simulink subsystem "aerodynamics"  (R2024b)
settings: Solver=VariableStepAuto  StartTime=0.0  StopTime=10.0  RelTol=1e-3
undefined symbols (not defined in the file): aero1d__ca0__mach, aero1d__ca0b__mach, aero1d__cad__mach, aero1d__cllp__mach, aero1d__clmq__mach, aero1d__clnr__mach, aero3d__caa__mach__alpha__beta, aero3d__cll0__mach__alpha__beta, aero3d__clldp__mach__alpha__beta, aero3d__clm0__mach__alpha__beta, aero3d__clmdq__mach__alpha__beta, aero3d__cln0__mach__alpha__beta, aero3d__clndr__mach__alpha__beta, aero3d__cn0__mach__alpha__beta, aero3d__cndq__mach__alpha__beta, aero3d__cy0__mach__alpha__beta, aero3d__cydr__mach__alpha__beta, alpha_grid, beta_grid, mach_grid, refa, refl, xcg_ref
settings Model: Creator=yagiz  LastModifiedBy=yagiz

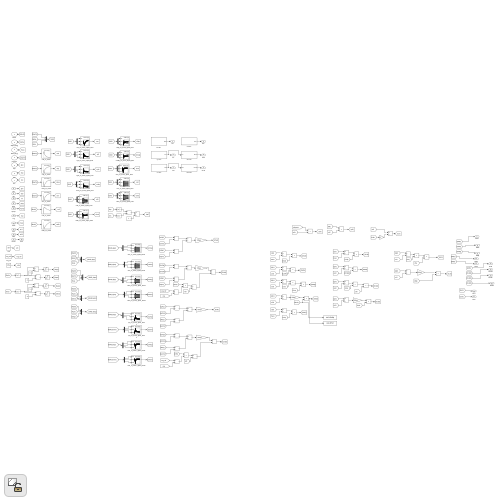
[thumbnail: Simulink's stored preview of the top-level diagram]
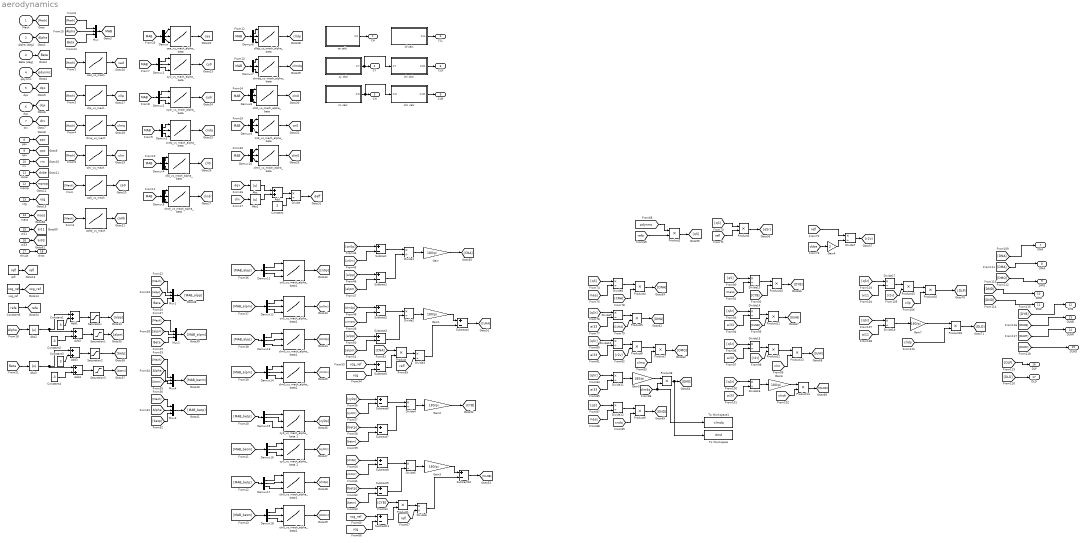
== system aerodynamics ==
  Mach : Inport
  Alpha [deg] : Inport  Port=2
  Beta [deg] : Inport  Port=3
  pdynmc : Inport  Port=4
  dpx : Inport  Port=5
  dqx : Inport  Port=6
  drx : Inport  Port=7
  ppx : Inport  Port=8
  qqx : Inport  Port=9
  rrx : Inport  Port=10
  dvbe : Inport  Port=11
  mprop : Inport  Port=12
  xcg : Inport  Port=13
  mass : Inport  Port=14
  ai11 : Inport  Port=15
  ai33 : Inport  Port=16
  thrust : Inport  Port=17
  Abs{,1..3} (4 alike) : Abs  SaturateOnIntegerOverflow=off
  Add{,1..4} (5 alike) : Sum
  Constant : Constant  Value=2
  Constant1 : Constant  Value=3
  Constant2 : Constant  Value=-3
  Constant3 : Constant  Value=3
  Constant4 : Constant  Value=-3
  Constant6 : Constant  Value=refa
  Demux{,1..18} (19 alike) : Demux  Outputs=3
  Divide{,1..18} (19 alike) : Product  Inputs=*/
  Gain{,1..3,5..7} (7 alike) : Gain  Gain=180/pi
  Gain4 : Gain  Gain=2
  Mux{,1..4} (5 alike) : Mux  Inputs=3
  Product{,1..16,18} (18 alike) : Product
  Saturation : Saturate  UpperLimit=inf  LowerLimit=3
  Saturation1 : Saturate  UpperLimit=inf  LowerLimit=0
  Saturation2 : Saturate  UpperLimit=inf  LowerLimit=3
  Saturation3 : Saturate  UpperLimit=inf  LowerLimit=0
  Subtract{,1..11} (12 alike) : Sum  Inputs=+-
  To Workspace : ToWorkspace  VariableName=dmd  SaveFormat=Timeseries  SampleTime=-1
  To Workspace1 : ToWorkspace  VariableName=clmdq  SaveFormat=Timeseries  SampleTime=-1
  ca calc : Subsystem
  ca0_vs_mach : Lookup_n-D  NumberOfTableDimensions=1  BreakpointsForDimension1=mach_grid  Table=aero1d__ca0__mach  InternalRulePriority=Speed  RndMeth=Simplest
  ca0b_vs_mach : Lookup_n-D  NumberOfTableDimensions=1  BreakpointsForDimension1=mach_grid  Table=aero1d__ca0b__mach  InternalRulePriority=Speed  RndMeth=Simplest
  caa_vs_mach_alpha_beta : Lookup_n-D  NumberOfTableDimensions=3  BreakpointsForDimension1=mach_grid  BreakpointsForDimension2=alpha_grid  BreakpointsForDimension3=beta_grid  Table=aero3d__caa__mach__alpha__beta  InternalRulePriority=Speed  RndMeth=Simplest
      settings: InputPortMap=u0,u1,u2
  cad_vs_mach : Lookup_n-D  NumberOfTableDimensions=1  BreakpointsForDimension1=mach_grid  Table=aero1d__cad__mach  InternalRulePriority=Speed  RndMeth=Simplest
  cll calc : Subsystem
  cll0_vs_mach_alpha_beta : Lookup_n-D  NumberOfTableDimensions=3  BreakpointsForDimension1=mach_grid  BreakpointsForDimension2=alpha_grid  BreakpointsForDimension3=beta_grid  Table=aero3d__cll0__mach__alpha__beta  InternalRulePriority=Speed  RndMeth=Simplest
      settings: InputPortMap=u0,u1,u2
  clldp_vs_mach_alpha_beta : Lookup_n-D  NumberOfTableDimensions=3  BreakpointsForDimension1=mach_grid  BreakpointsForDimension2=alpha_grid  BreakpointsForDimension3=beta_grid  Table=aero3d__clldp__mach__alpha__beta  InternalRulePriority=Speed  RndMeth=Simplest
      settings: InputPortMap=u0,u1,u2
  cllp_vs_mach : Lookup_n-D  NumberOfTableDimensions=1  BreakpointsForDimension1=mach_grid  Table=aero1d__cllp__mach  InternalRulePriority=Speed  RndMeth=Simplest
  clm calc : Subsystem
  clm0_vs_mach_alpha_beta : Lookup_n-D  NumberOfTableDimensions=3  BreakpointsForDimension1=mach_grid  BreakpointsForDimension2=alpha_grid  BreakpointsForDimension3=beta_grid  Table=aero3d__clm0__mach__alpha__beta  InternalRulePriority=Speed  RndMeth=Simplest
      settings: InputPortMap=u0,u1,u2
  clm0_vs_mach_alpha_beta1 : Lookup_n-D  NumberOfTableDimensions=3  BreakpointsForDimension1=mach_grid  BreakpointsForDimension2=alpha_grid  BreakpointsForDimension3=beta_grid  Table=aero3d__clm0__mach__alpha__beta  InternalRulePriority=Speed  RndMeth=Simplest
      settings: InputPortMap=u0,u1,u2
  clm0_vs_mach_alpha_beta2 : Lookup_n-D  NumberOfTableDimensions=3  BreakpointsForDimension1=mach_grid  BreakpointsForDimension2=alpha_grid  BreakpointsForDimension3=beta_grid  Table=aero3d__clm0__mach__alpha__beta  InternalRulePriority=Speed  RndMeth=Simplest
      settings: InputPortMap=u0,u1,u2
  clmdq_vs_mach_alpha_beta : Lookup_n-D  NumberOfTableDimensions=3  BreakpointsForDimension1=mach_grid  BreakpointsForDimension2=alpha_grid  BreakpointsForDimension3=beta_grid  Table=aero3d__clmdq__mach__alpha__beta  InternalRulePriority=Speed  RndMeth=Simplest
      settings: InputPortMap=u0,u1,u2
  clmq_vs_mach : Lookup_n-D  NumberOfTableDimensions=1  BreakpointsForDimension1=mach_grid  Table=aero1d__clmq__mach  InternalRulePriority=Speed  RndMeth=Simplest
  cln calc : Subsystem
  cln0_vs_mach_alpha_beta : Lookup_n-D  NumberOfTableDimensions=3  BreakpointsForDimension1=mach_grid  BreakpointsForDimension2=alpha_grid  BreakpointsForDimension3=beta_grid  Table=aero3d__cln0__mach__alpha__beta  InternalRulePriority=Speed  RndMeth=Simplest
      settings: InputPortMap=u0,u1,u2
  cln0_vs_mach_alpha_beta1 : Lookup_n-D  NumberOfTableDimensions=3  BreakpointsForDimension1=mach_grid  BreakpointsForDimension2=alpha_grid  BreakpointsForDimension3=beta_grid  Table=aero3d__cln0__mach__alpha__beta  InternalRulePriority=Speed  RndMeth=Simplest
      settings: InputPortMap=u0,u1,u2
  cln0_vs_mach_alpha_beta2 : Lookup_n-D  NumberOfTableDimensions=3  BreakpointsForDimension1=mach_grid  BreakpointsForDimension2=alpha_grid  BreakpointsForDimension3=beta_grid  Table=aero3d__cln0__mach__alpha__beta  InternalRulePriority=Speed  RndMeth=Simplest
      settings: InputPortMap=u0,u1,u2
  "clndr_vs_mach_alpha_beta " : Lookup_n-D  NumberOfTableDimensions=3  BreakpointsForDimension1=mach_grid  BreakpointsForDimension2=alpha_grid  BreakpointsForDimension3=beta_grid  Table=aero3d__clndr__mach__alpha__beta  InternalRulePriority=Speed  RndMeth=Simplest
      settings: InputPortMap=u0,u1,u2
  clnr_vs_mach : Lookup_n-D  NumberOfTableDimensions=1  BreakpointsForDimension1=mach_grid  Table=aero1d__clnr__mach  InternalRulePriority=Speed  RndMeth=Simplest
  cn calc : Subsystem
  cn0_vs_mach_alpha_beta : Lookup_n-D  NumberOfTableDimensions=3  BreakpointsForDimension1=mach_grid  BreakpointsForDimension2=alpha_grid  BreakpointsForDimension3=beta_grid  Table=aero3d__cn0__mach__alpha__beta  InternalRulePriority=Speed  RndMeth=Simplest
      settings: InputPortMap=u0,u1,u2
  cn0_vs_mach_alpha_beta1 : Lookup_n-D  NumberOfTableDimensions=3  BreakpointsForDimension1=mach_grid  BreakpointsForDimension2=alpha_grid  BreakpointsForDimension3=beta_grid  Table=aero3d__cn0__mach__alpha__beta  InternalRulePriority=Speed  RndMeth=Simplest
      settings: InputPortMap=u0,u1,u2
  cn0_vs_mach_alpha_beta2 : Lookup_n-D  NumberOfTableDimensions=3  BreakpointsForDimension1=mach_grid  BreakpointsForDimension2=alpha_grid  BreakpointsForDimension3=beta_grid  Table=aero3d__cn0__mach__alpha__beta  InternalRulePriority=Speed  RndMeth=Simplest
      settings: InputPortMap=u0,u1,u2
  cndq_vs_mach_alpha_beta : Lookup_n-D  NumberOfTableDimensions=3  BreakpointsForDimension1=mach_grid  BreakpointsForDimension2=alpha_grid  BreakpointsForDimension3=beta_grid  Table=aero3d__cndq__mach__alpha__beta  InternalRulePriority=Speed  RndMeth=Simplest
      settings: InputPortMap=u0,u1,u2
  cy calc : Subsystem
  "cy0_vs_mach_alpha_beta " : Lookup_n-D  NumberOfTableDimensions=3  BreakpointsForDimension1=mach_grid  BreakpointsForDimension2=alpha_grid  BreakpointsForDimension3=beta_grid  Table=aero3d__cy0__mach__alpha__beta  InternalRulePriority=Speed  RndMeth=Simplest
      settings: InputPortMap=u0,u1,u2
  cy0_vs_mach_alpha_beta 1 : Lookup_n-D  NumberOfTableDimensions=3  BreakpointsForDimension1=mach_grid  BreakpointsForDimension2=alpha_grid  BreakpointsForDimension3=beta_grid  Table=aero3d__cy0__mach__alpha__beta  InternalRulePriority=Speed  RndMeth=Simplest
      settings: InputPortMap=u0,u1,u2
  cy0_vs_mach_alpha_beta 2 : Lookup_n-D  NumberOfTableDimensions=3  BreakpointsForDimension1=mach_grid  BreakpointsForDimension2=alpha_grid  BreakpointsForDimension3=beta_grid  Table=aero3d__cy0__mach__alpha__beta  InternalRulePriority=Speed  RndMeth=Simplest
      settings: InputPortMap=u0,u1,u2
  cydr_vs_mach_alpha_beta : Lookup_n-D  NumberOfTableDimensions=3  BreakpointsForDimension1=mach_grid  BreakpointsForDimension2=alpha_grid  BreakpointsForDimension3=beta_grid  Table=aero3d__cydr__mach__alpha__beta  InternalRulePriority=Speed  RndMeth=Simplest
      settings: InputPortMap=u0,u1,u2
  refl : Constant  Value=refl
  xcg_ref : Constant  Value=xcg_ref
  CA : Outport
  CY : Outport  Port=2
  CN : Outport  Port=3
  CLL : Outport  Port=4
  CLM : Outport  Port=5
  CLN : Outport  Port=6
  DNA : Outport  Port=7
  DMA : Outport  Port=8
  DMQ : Outport  Port=9
  DMD : Outport  Port=10
  DND : Outport  Port=11
  DYB : Outport  Port=12
  DLNB : Outport  Port=13
  DLNR : Outport  Port=14
  DLND : Outport  Port=15
  DLP : Outport  Port=16
  DLD : Outport  Port=17
  thrst : Outport  Port=18
  tag scope: Alpha=global, Beta=global, MAB=global, ai11=global, ai33=global, ca0=global, ca0b=global, caa=global, cad=global, cll0=global, clldp=global, cllp=global, clm0=global, clmdq=global, clmq=global, cln0=global, clndr=global, clnr=global, cn0=global, cndq=global, cy0=global, cydr=global, deff=global, dpx=global, dqx=global, drx=global, dvbe=global, mass=global, mprop=global, pdynmc=global, ppx=global, qqx=global, refa=global, refl=global, rrx=global, xcg=global, xcg_ref=global
  wires:
  Mach/1 -> [Mach]
  Alpha [deg]/1 -> [Alpha]
  Beta [deg]/1 -> [Beta]
  [Mach] -> ca0_vs_mach/1
  [Mach] -> ca0b_vs_mach/1
  [Mach] -> cad_vs_mach/1
  [Mach] -> cllp_vs_mach/1
  [Mach] -> clmq_vs_mach/1
  [Mach] -> clnr_vs_mach/1
  [Alpha] -> Mux/2
  [Mach] -> Mux/1
  [Beta] -> Mux/3
  Mux/1 -> [MAB]
  [MAB] -> Demux/1
  Demux/1 -> caa_vs_mach_alpha_beta/1
  Demux/2 -> caa_vs_mach_alpha_beta/2
  Demux/3 -> caa_vs_mach_alpha_beta/3
  [MAB] -> Demux1/1
  Demux1/2 -> "cy0_vs_mach_alpha_beta "/2
  Demux1/1 -> "cy0_vs_mach_alpha_beta "/1
  Demux1/3 -> "cy0_vs_mach_alpha_beta "/3
  [MAB] -> Demux2/1
  Demux2/2 -> cydr_vs_mach_alpha_beta/2
  Demux2/1 -> cydr_vs_mach_alpha_beta/1
  Demux2/3 -> cydr_vs_mach_alpha_beta/3
  [MAB] -> Demux3/1
  Demux3/2 -> cndq_vs_mach_alpha_beta/2
  Demux3/1 -> cndq_vs_mach_alpha_beta/1
  Demux3/3 -> cndq_vs_mach_alpha_beta/3
  [MAB] -> Demux4/1
  Demux4/2 -> cll0_vs_mach_alpha_beta/2
  Demux4/1 -> cll0_vs_mach_alpha_beta/1
  Demux4/3 -> cll0_vs_mach_alpha_beta/3
  [MAB] -> Demux5/1
  Demux5/2 -> "clndr_vs_mach_alpha_beta "/2
  Demux5/1 -> "clndr_vs_mach_alpha_beta "/1
  Demux5/3 -> "clndr_vs_mach_alpha_beta "/3
  [MAB] -> Demux6/1
  Demux6/2 -> clldp_vs_mach_alpha_beta/2
  Demux6/1 -> clldp_vs_mach_alpha_beta/1
  Demux6/3 -> clldp_vs_mach_alpha_beta/3
  [MAB] -> Demux7/1
  Demux7/2 -> clmdq_vs_mach_alpha_beta/2
  Demux7/1 -> clmdq_vs_mach_alpha_beta/1
  Demux7/3 -> clmdq_vs_mach_alpha_beta/3
  [MAB] -> Demux8/1
  Demux8/2 -> cln0_vs_mach_alpha_beta/2
  Demux8/1 -> cln0_vs_mach_alpha_beta/1
  Demux8/3 -> cln0_vs_mach_alpha_beta/3
  pdynmc/1 -> [pdynmc]
  dpx/1 -> [dpx]
  dqx/1 -> [dqx]
  drx/1 -> [drx]
  qqx/1 -> [qqx]
  ppx/1 -> [ppx]
  rrx/1 -> [rrx]
  dvbe/1 -> [dvbe]
  mprop/1 -> [mprop]
  refl/1 -> [refl]
  xcg_ref/1 -> [xcg_ref]
  xcg/1 -> [xcg]
  cad_vs_mach/1 -> [cad]
  cllp_vs_mach/1 -> [cllp]
  clmq_vs_mach/1 -> [clmq]
  clnr_vs_mach/1 -> [clnr]
  ca0_vs_mach/1 -> [ca0]
  ca0b_vs_mach/1 -> [ca0b]
  caa_vs_mach_alpha_beta/1 -> [caa]
  "cy0_vs_mach_alpha_beta "/1 -> [cy0]
  cydr_vs_mach_alpha_beta/1 -> [cydr]
  cndq_vs_mach_alpha_beta/1 -> [cndq]
  cll0_vs_mach_alpha_beta/1 -> [cll0]
  "clndr_vs_mach_alpha_beta "/1 -> [clndr]
  clldp_vs_mach_alpha_beta/1 -> [clldp]
  clmdq_vs_mach_alpha_beta/1 -> [clmdq]
  cln0_vs_mach_alpha_beta/1 -> [cln0]
  [dqx] -> Abs/1
  Abs/1 -> Add/1
  Abs1/1 -> Add/2
  [drx] -> Abs1/1
  Add/1 -> Divide/1
  Constant/1 -> Divide/2
  Divide/1 -> [deff]
  [MAB] -> Demux9/1
  Demux9/2 -> cn0_vs_mach_alpha_beta/2
  cn0_vs_mach_alpha_beta/1 -> [cn0]
  Demux9/1 -> cn0_vs_mach_alpha_beta/1
  Demux9/3 -> cn0_vs_mach_alpha_beta/3
  Demux10/2 -> clm0_vs_mach_alpha_beta/2
  clm0_vs_mach_alpha_beta/1 -> [clm0]
  Demux10/3 -> clm0_vs_mach_alpha_beta/3
  Demux10/1 -> clm0_vs_mach_alpha_beta/1
  [MAB] -> Demux10/1
  ca calc/1(CA) -> CA/1
  cy calc/1(CY) -> cln calc/1(CY), CY/1
  cn calc/1(CN) -> clm calc/1(CN), CN/1
  cll calc/1(CLL) -> CLL/1
  clm calc/1(CLM) -> CLM/1
  cln calc/1(CLN) -> CLN/1
  [Alpha] -> Abs2/1
  Abs2/1 -> Add2/1, Add1/1
  Constant1/1 -> Add1/2
  Add1/1 -> Saturation/1
  Saturation/1 -> [alpp]
  Add2/1 -> Saturation1/1
  Saturation1/1 -> [alpm]
  Constant2/1 -> Add2/2
  [Beta] -> Abs3/1
  Saturation2/1 -> [betp]
  Add3/1 -> Saturation2/1
  Abs3/1 -> Add4/1, Add3/1
  Saturation3/1 -> [betm]
  Add4/1 -> Saturation3/1
  Constant4/1 -> Add4/2
  Constant3/1 -> Add3/2
  [Mach] -> Mux1/1
  [alpp] -> Mux1/2
  [Beta] -> Mux1/3
  [Beta] -> Mux2/3
  [Mach] -> Mux2/1
  [alpm] -> Mux2/2
  [betp] -> Mux3/3
  [Mach] -> Mux3/1
  [Alpha] -> Mux3/2
  [Mach] -> Mux4/1
  [Alpha] -> Mux4/2
  [betm] -> Mux4/3
  Mux1/1 -> [MAB_alpp]
  Mux2/1 -> [MAB_alpm]
  Mux4/1 -> [MAB_betm]
  Mux3/1 -> [MAB_betp]
  [MAB_alpp] -> Demux11/1
  Demux11/1 -> cn0_vs_mach_alpha_beta1/1
  Demux11/2 -> cn0_vs_mach_alpha_beta1/2
  Demux11/3 -> cn0_vs_mach_alpha_beta1/3
  Demux12/1 -> cn0_vs_mach_alpha_beta2/1
  Demux12/2 -> cn0_vs_mach_alpha_beta2/2
  [MAB_alpm] -> Demux12/1
  Demux12/3 -> cn0_vs_mach_alpha_beta2/3
  Demux14/1 -> clm0_vs_mach_alpha_beta2/1
  Demux13/1 -> clm0_vs_mach_alpha_beta1/1
  Demux13/2 -> clm0_vs_mach_alpha_beta1/2
  Demux14/3 -> clm0_vs_mach_alpha_beta2/3
  [MAB_alpm] -> Demux14/1
  Demux14/2 -> clm0_vs_mach_alpha_beta2/2
  [MAB_alpp] -> Demux13/1
  Demux13/3 -> clm0_vs_mach_alpha_beta1/3
  cn0_vs_mach_alpha_beta1/1 -> [cn0p]
  cn0_vs_mach_alpha_beta2/1 -> [cn0m]
  clm0_vs_mach_alpha_beta1/1 -> [clm0p]
  clm0_vs_mach_alpha_beta2/1 -> [clm0m]
  Demux17/1 -> cln0_vs_mach_alpha_beta1/1
  Demux16/2 -> cy0_vs_mach_alpha_beta 2/2
  Demux18/1 -> cln0_vs_mach_alpha_beta2/1
  Demux18/2 -> cln0_vs_mach_alpha_beta2/2
  Demux18/3 -> cln0_vs_mach_alpha_beta2/3
  Demux17/2 -> cln0_vs_mach_alpha_beta1/2
  Demux15/3 -> cy0_vs_mach_alpha_beta 1/3
  [MAB_betm] -> Demux16/1
  Demux16/3 -> cy0_vs_mach_alpha_beta 2/3
  Demux15/2 -> cy0_vs_mach_alpha_beta 1/2
  Demux15/1 -> cy0_vs_mach_alpha_beta 1/1
  Demux17/3 -> cln0_vs_mach_alpha_beta1/3
  [MAB_betp] -> Demux15/1
  Demux16/1 -> cy0_vs_mach_alpha_beta 2/1
  [MAB_betm] -> Demux18/1
  [MAB_betp] -> Demux17/1
  cy0_vs_mach_alpha_beta 1/1 -> [cy0p]
  cy0_vs_mach_alpha_beta 2/1 -> [cy0m]
  cln0_vs_mach_alpha_beta1/1 -> [cln0p]
  cln0_vs_mach_alpha_beta2/1 -> [cln0m]
  [cn0p] -> Subtract/1
  [cn0m] -> Subtract/2
  Subtract/1 -> Divide1/1
  [alpm] -> Subtract1/2
  [alpp] -> Subtract1/1
  Subtract1/1 -> Divide1/2
  Divide1/1 -> Gain/1
  Gain/1 -> [CNA]
  Divide2/1 -> Gain1/1
  Subtract3/1 -> Divide2/2
  [alpm] -> Subtract3/2
  [alpp] -> Subtract3/1
  [clm0m] -> Subtract2/2
  Subtract2/1 -> Divide2/1
  [clm0p] -> Subtract2/1
  Gain1/1 -> Subtract4/1
  [CNA] -> Product/1
  Subtract5/1 -> Product/2
  [xcg_ref] -> Subtract5/1
  [xcg] -> Subtract5/2
  Product/1 -> Divide3/1
  [refl] -> Divide3/2
  Divide3/1 -> Subtract4/2
  Subtract4/1 -> [CLMA]
  Divide4/1 -> Gain2/1
  Subtract7/1 -> Divide4/2
  [betm] -> Subtract7/2
  [betp] -> Subtract7/1
  [cy0m] -> Subtract6/2
  Subtract6/1 -> Divide4/1
  [cy0p] -> Subtract6/1
  Gain2/1 -> [CYB]
  [cln0m] -> Subtract8/2
  Subtract10/1 -> [CLNB]
  Divide6/1 -> Subtract10/2
  Divide5/1 -> Gain3/1
  [xcg] -> Subtract11/2
  Subtract11/1 -> Product1/2
  Product1/1 -> Divide6/1
  [xcg_ref] -> Subtract11/1
  [CYB] -> Product1/1
  Subtract8/1 -> Divide5/1
  [betp] -> Subtract9/1
  [refl] -> Divide6/2
  [betm] -> Subtract9/2
  [cln0p] -> Subtract8/1
  Subtract9/1 -> Divide5/2
  Gain3/1 -> Subtract10/1
  [pdynmc] -> Product2/1
  [refa] -> Product2/2
  Constant6/1 -> [refa]
  Product2/1 -> [qS]
  [qS] -> Product3/1
  [refl] -> Product3/2
  Product3/1 -> [qSr]
  [refl] -> Divide7/1
  [dvbe] -> Gain4/1
  Gain4/1 -> Divide7/2
  Divide7/1 -> [r2v]
  [qS] -> Divide8/1
  mass/1 -> [mass]
  [mass] -> Divide8/2
  Divide8/1 -> Product4/1
  Product4/1 -> [DNA]
  ai11/1 -> [ai11]
  ai33/1 -> [ai33]
  Product5/1 -> [DMA]
  [qSr] -> Divide9/1
  Divide9/1 -> Product5/1
  [ai33] -> Divide9/2
  [CNA] -> Product4/2
  [CLMA] -> Product5/2
  Product6/1 -> Product7/1
  [r2v] -> Product6/2
  Divide10/1 -> Product6/1
  [qSr] -> Divide10/1
  [ai33] -> Divide10/2
  [clmq] -> Product7/2
  Product7/1 -> [DMQ]
  Divide11/1 -> Gain5/1
  [qSr] -> Divide11/1
  [ai33] -> Divide11/2
  Gain5/1 -> Product8/1
  [clmdq] -> Product8/2, To Workspace1/1
  Product8/1 -> [DMD], To Workspace/1
  [cndq] -> Product9/2
  [qS] -> Divide12/1
  [mass] -> Divide12/2
  Divide12/1 -> Product9/1
  Product9/1 -> [DND]
  [CYB] -> Product10/2
  [qS] -> Divide13/1
  [mass] -> Divide13/2
  Divide13/1 -> Product10/1
  Product10/1 -> [DYB]
  Product11/1 -> [DLNB]
  [CLNB] -> Product11/2
  Divide14/1 -> Product11/1
  [qSr] -> Divide14/1
  [ai33] -> Divide14/2
  [r2v] -> Product12/2
  Product12/1 -> Product13/1
  [clnr] -> Product13/2
  [qSr] -> Divide15/1
  [ai33] -> Divide15/2
  Divide15/1 -> Product12/1
  Product13/1 -> [DLNR]
  [qSr] -> Divide16/1
  Gain6/1 -> Product14/1
  [clndr] -> Product14/2
  Product14/1 -> [DLND]
  [ai33] -> Divide16/2
  Divide16/1 -> Gain6/1
  Product15/1 -> Product16/1
  [r2v] -> Product15/2
  Divide17/1 -> Product15/1
  [qSr] -> Divide17/1
  [ai11] -> Divide17/2
  [cllp] -> Product16/2
  [qSr] -> Divide18/1
  [clldp] -> Product18/2
  Gain7/1 -> Product18/1
  Product18/1 -> [DLD]
  [ai11] -> Divide18/2
  Divide18/1 -> Gain7/1
  [DNA] -> DNA/1
  [DMA] -> DMA/1
  [DMQ] -> DMQ/1
  [DMD] -> DMD/1
  [DND] -> DND/1
  [DYB] -> DYB/1
  [DLNB] -> DLNB/1
  [DLNR] -> DLNR/1
  [DLND] -> DLND/1
  [DLP] -> DLP/1
  [DLD] -> DLD/1
  thrust/1 -> thrst/1
  Product16/1 -> [DLP]

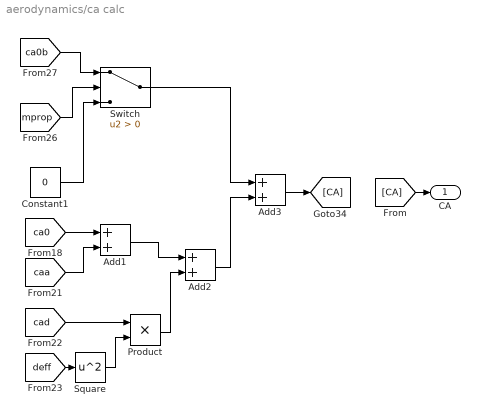
== system aerodynamics/ca calc ==
  Add1 : Sum
  Add2 : Sum
  Add3 : Sum
  Constant1 : Constant  Value=0
  Product : Product
  Square : Math  Operator=square
  Switch : Switch  Criteria=u2 > Threshold  SaturateOnIntegerOverflow=off  InputSameDT=off
  CA : Outport
  wires:
  [ca0] -> Add1/1
  Add3/1 -> [CA]
  [caa] -> Add1/2
  Square/1 -> Product/2
  [mprop] -> Switch/2
  [cad] -> Product/1
  Constant1/1 -> Switch/3
  [ca0b] -> Switch/1
  [deff] -> Square/1
  Add1/1 -> Add2/1
  Switch/1 -> Add3/1
  Add2/1 -> Add3/2
  Product/1 -> Add2/2
  [CA] -> CA/1

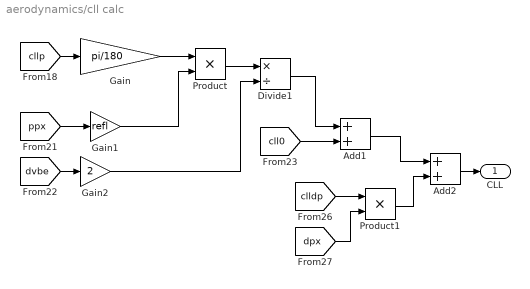
== system aerodynamics/cll calc ==
  Add1 : Sum
  Add2 : Sum
  Divide1 : Product  Inputs=*/
  Gain : Gain  Gain=pi/180
  Gain1 : Gain  Gain=refl
  Gain2 : Gain  Gain=2
  Product : Product
  Product1 : Product
  CLL : Outport
  wires:
  [ppx] -> Gain1/1
  Add2/1 -> CLL/1
  Divide1/1 -> Add1/1
  Product1/1 -> Add2/2
  [dpx] -> Product1/2
  Gain2/1 -> Divide1/2
  [dvbe] -> Gain2/1
  Gain1/1 -> Product/2
  Gain/1 -> Product/1
  Product/1 -> Divide1/1
  [cll0] -> Add1/2
  Add1/1 -> Add2/1
  [clldp] -> Product1/1
  [cllp] -> Gain/1

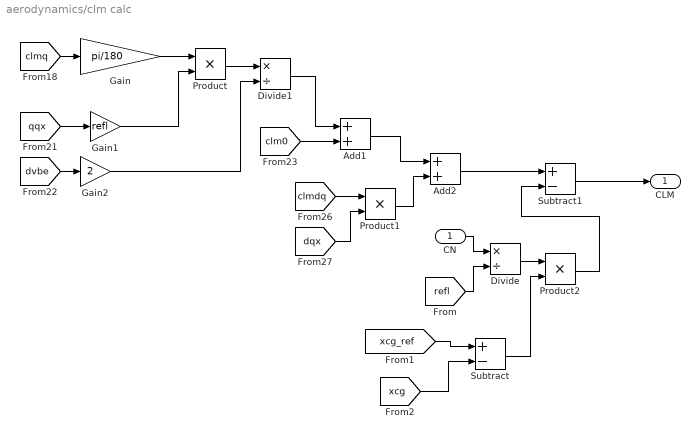
== system aerodynamics/clm calc ==
  CN : Inport
  Add1 : Sum
  Add2 : Sum
  Divide : Product  Inputs=*/
  Divide1 : Product  Inputs=*/
  Gain : Gain  Gain=pi/180
  Gain1 : Gain  Gain=refl
  Gain2 : Gain  Gain=2
  Product : Product
  Product1 : Product
  Product2 : Product
  Subtract : Sum  Inputs=+-
  Subtract1 : Sum  Inputs=+-
  CLM : Outport
  wires:
  [qqx] -> Gain1/1
  Divide1/1 -> Add1/1
  Product1/1 -> Add2/2
  [dqx] -> Product1/2
  Gain2/1 -> Divide1/2
  [dvbe] -> Gain2/1
  Gain1/1 -> Product/2
  Gain/1 -> Product/1
  Product/1 -> Divide1/1
  [clm0] -> Add1/2
  Add1/1 -> Add2/1
  [clmdq] -> Product1/1
  [clmq] -> Gain/1
  CN/1 -> Divide/1
  [refl] -> Divide/2
  Divide/1 -> Product2/1
  [xcg_ref] -> Subtract/1
  [xcg] -> Subtract/2
  Subtract/1 -> Product2/2
  Add2/1 -> Subtract1/1
  Product2/1 -> Subtract1/2
  Subtract1/1 -> CLM/1

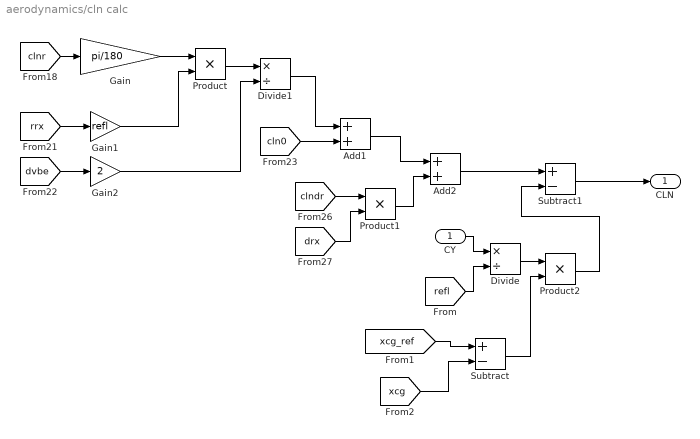
== system aerodynamics/cln calc ==
  CY : Inport
  Add1 : Sum
  Add2 : Sum
  Divide : Product  Inputs=*/
  Divide1 : Product  Inputs=*/
  Gain : Gain  Gain=pi/180
  Gain1 : Gain  Gain=refl
  Gain2 : Gain  Gain=2
  Product : Product
  Product1 : Product
  Product2 : Product
  Subtract : Sum  Inputs=+-
  Subtract1 : Sum  Inputs=+-
  CLN : Outport
  wires:
  [rrx] -> Gain1/1
  Divide1/1 -> Add1/1
  Product1/1 -> Add2/2
  [drx] -> Product1/2
  Gain2/1 -> Divide1/2
  [dvbe] -> Gain2/1
  Gain1/1 -> Product/2
  Gain/1 -> Product/1
  Product/1 -> Divide1/1
  [cln0] -> Add1/2
  Add1/1 -> Add2/1
  [clndr] -> Product1/1
  [clnr] -> Gain/1
  CY/1 -> Divide/1
  [refl] -> Divide/2
  Divide/1 -> Product2/1
  [xcg_ref] -> Subtract/1
  [xcg] -> Subtract/2
  Subtract/1 -> Product2/2
  Add2/1 -> Subtract1/1
  Product2/1 -> Subtract1/2
  Subtract1/1 -> CLN/1

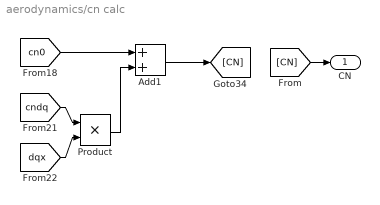
== system aerodynamics/cn calc ==
  Add1 : Sum
  Product : Product
  CN : Outport
  wires:
  [dqx] -> Product/2
  Add1/1 -> [CN]
  [cndq] -> Product/1
  [cn0] -> Add1/1
  Product/1 -> Add1/2
  [CN] -> CN/1

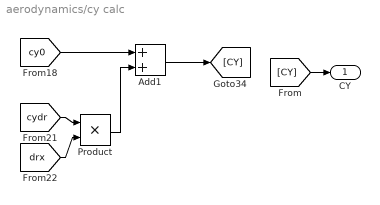
== system aerodynamics/cy calc ==
  Add1 : Sum
  Product : Product
  CY : Outport
  wires:
  [drx] -> Product/2
  Add1/1 -> [CY]
  [cydr] -> Product/1
  [cy0] -> Add1/1
  Product/1 -> Add1/2
  [CY] -> CY/1
